simulink library "sf_aircraft_screen_library"  (Simulink 7.6)
settings: Solver=ode45  SolverMode=SingleTasking  StartTime=0.0  StopTime=10.0  RelTol=1e-3
settings Model: Creator=The MathWorks Inc.

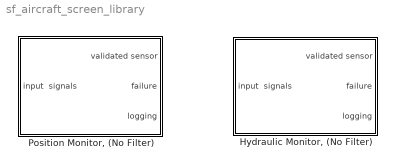
== system sf_aircraft_screen_library ==
  "Hydraulic Monitor, (No Filter)" : Subsystem  AncestorBlock=screen_library/Hydraulic Monitor
  "Position Monitor, (No Filter)" : Subsystem

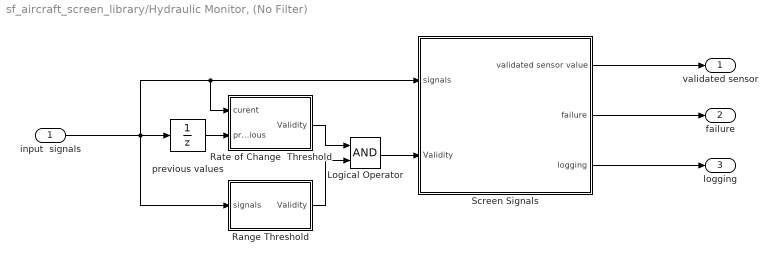
== system sf_aircraft_screen_library/Hydraulic Monitor, (No Filter) ==
  input  signals : Inport  PortDimensions=3  SampleTime=0.01
  Logical Operator : Logic  AllPortsSameDT=off
  Range Threshold : Subsystem
  Rate of Change  Threshold : Subsystem
  Screen Signals : Subsystem
  previous values : UnitDelay  SampleTime=-1
  validated sensor : Outport
  failure : Outport  Port=2
  logging : Outport  Port=3
  wires:
  Screen Signals/3(logging) -> logging/1
  Logical Operator/1 -> Screen Signals/2(Validity)
  Rate of Change  Threshold/1(Validity) -> Logical Operator/1
  Range Threshold/1(Validity) -> Logical Operator/2
  previous values/1 -> Rate of Change  Threshold/2(previous)
  Screen Signals/1(validated sensor value) -> validated sensor/1
  input  signals/1 -> Range Threshold/1(signals), Screen Signals/1(signals), Rate of Change  Threshold/1(curent), previous values/1
  Screen Signals/2(failure) -> failure/1

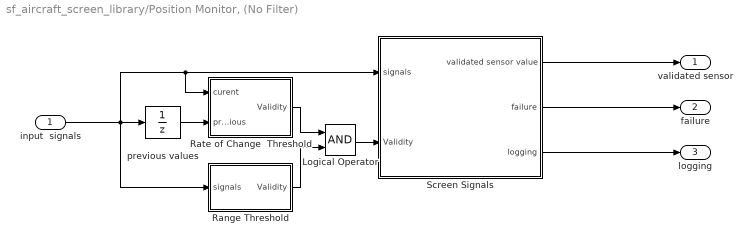
== system sf_aircraft_screen_library/Position Monitor, (No Filter) ==
  input  signals : Inport  PortDimensions=3  SampleTime=0.01
  Logical Operator : Logic  AllPortsSameDT=off
  Range Threshold : Subsystem  RequirementInfo={'other' 'Position Sensor Logic Requirements.doc' 'Out of Bound Readings' 'true' 'Out of Bound Readings' '' }
  Rate of Change  Threshold : Subsystem  RequirementInfo={'other' 'Position Sensor Logic Requirements.doc' 'Rate of Change of Readings' 'true' 'Rate of Change of Readings' '' }
  Screen Signals : Subsystem
  previous values : UnitDelay  SampleTime=-1
  validated sensor : Outport
  failure : Outport  Port=2
  logging : Outport  Port=3
  wires:
  Screen Signals/3(logging) -> logging/1
  Screen Signals/2(failure) -> failure/1
  input  signals/1 -> Range Threshold/1(signals), previous values/1, Screen Signals/1(signals), Rate of Change  Threshold/1(curent)
  Screen Signals/1(validated sensor value) -> validated sensor/1
  previous values/1 -> Rate of Change  Threshold/2(previous)
  Range Threshold/1(Validity) -> Logical Operator/2
  Rate of Change  Threshold/1(Validity) -> Logical Operator/1
  Logical Operator/1 -> Screen Signals/2(Validity)

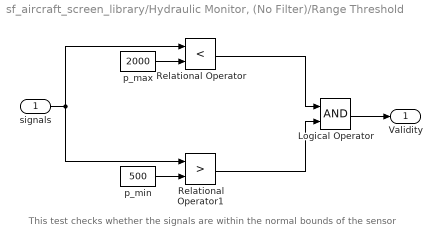
== system sf_aircraft_screen_library/Hydraulic Monitor, (No Filter)/Range Threshold ==
  note: This test checks whether the signals are within
      | the normal bounds of the sensor
  signals : Inport
  Logical Operator : Logic  AllPortsSameDT=off
  Relational Operator : RelationalOperator  Operator=<
  Relational Operator1 : RelationalOperator  Operator=>
  p_max : Constant  Value=2000
  p_min : Constant  Value=500
  Validity : Outport
  wires:
  Logical Operator/1 -> Validity/1
  p_min/1 -> Relational Operator1/2
  p_max/1 -> Relational Operator/2
  Relational Operator1/1 -> Logical Operator/2
  Relational Operator/1 -> Logical Operator/1
  signals/1 -> Relational Operator1/1, Relational Operator/1

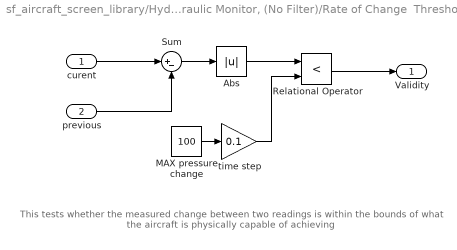
== system sf_aircraft_screen_library/Hydraulic Monitor, (No Filter)/Rate of Change  Threshold ==
  note: This tests whether the measured change between two readings
      | is within the bounds of what the aircraft is physically capable of achieving
  curent : Inport
  previous : Inport  Port=2
  Abs : Abs  SaturateOnIntegerOverflow=on
  MAX pressure change : Constant  Value=100
  Relational Operator : RelationalOperator  Operator=<  OutDataTypeStr=boolean
  Sum : Sum  Inputs=|+-  SaturateOnIntegerOverflow=on
  time step : Gain  Gain=0.1  SaturateOnIntegerOverflow=on  OutDataTypeStr=Inherit: Same as input  ParamDataTypeStr=Inherit: Same as input
  Validity : Outport
  wires:
  Sum/1 -> Abs/1
  time step/1 -> Relational Operator/2
  MAX pressure change/1 -> time step/1
  Relational Operator/1 -> Validity/1
  previous/1 -> Sum/2
  curent/1 -> Sum/1
  Abs/1 -> Relational Operator/1

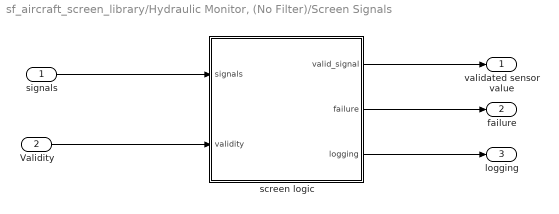
== system sf_aircraft_screen_library/Hydraulic Monitor, (No Filter)/Screen Signals ==
  signals : Inport
  Validity : Inport  Port=2
  screen logic : Stateflow chart  AncestorBlock=new_screening/Montior/Screen Signals/screen logic  TreatAsAtomicUnit=on
  validated sensor value : Outport
  failure : Outport  Port=2
  logging : Outport  Port=3
  wires:
  screen logic/3(logging) -> logging/1
  signals/1 -> screen logic/1(signals)
  Validity/1 -> screen logic/2(validity)
  screen logic/1(valid_signal) -> validated sensor value/1
  screen logic/2(failure) -> failure/1

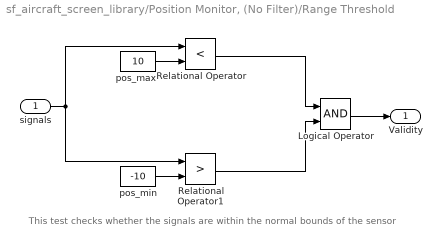
== system sf_aircraft_screen_library/Position Monitor, (No Filter)/Range Threshold ==
  note: This test checks whether the signals are within
      | the normal bounds of the sensor
  signals : Inport
  Logical Operator : Logic  AllPortsSameDT=off
  Relational Operator : RelationalOperator  Operator=<
  Relational Operator1 : RelationalOperator  Operator=>
  pos_max : Constant  Value=10
  pos_min : Constant  Value=-10
  Validity : Outport
  wires:
  Logical Operator/1 -> Validity/1
  pos_min/1 -> Relational Operator1/2
  pos_max/1 -> Relational Operator/2
  Relational Operator1/1 -> Logical Operator/2
  Relational Operator/1 -> Logical Operator/1
  signals/1 -> Relational Operator1/1, Relational Operator/1

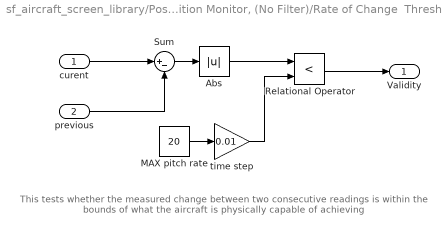
== system sf_aircraft_screen_library/Position Monitor, (No Filter)/Rate of Change  Threshold ==
  note: This tests whether the measured change between two consecutive readings
      | is within the bounds of what the aircraft is physically capable of achieving
  curent : Inport
  previous : Inport  Port=2
  Abs : Abs  SaturateOnIntegerOverflow=on
  MAX pitch rate : Constant  Value=20
  Relational Operator : RelationalOperator  Operator=<  OutDataTypeStr=boolean
  Sum : Sum  Inputs=|+-  SaturateOnIntegerOverflow=on
  time step : Gain  Gain=0.01  SaturateOnIntegerOverflow=on  OutDataTypeStr=Inherit: Same as input  ParamDataTypeStr=Inherit: Same as input
  Validity : Outport
  wires:
  curent/1 -> Sum/1
  previous/1 -> Sum/2
  Relational Operator/1 -> Validity/1
  MAX pitch rate/1 -> time step/1
  time step/1 -> Relational Operator/2
  Sum/1 -> Abs/1
  Abs/1 -> Relational Operator/1

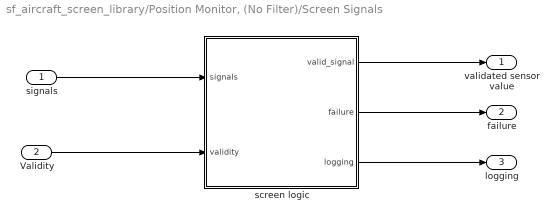
== system sf_aircraft_screen_library/Position Monitor, (No Filter)/Screen Signals ==
  signals : Inport
  Validity : Inport  Port=2
  screen logic : Stateflow chart  TreatAsAtomicUnit=on
  validated sensor value : Outport
  failure : Outport  Port=2
  logging : Outport  Port=3
  wires:
  screen logic/3(logging) -> logging/1
  screen logic/2(failure) -> failure/1
  screen logic/1(valid_signal) -> validated sensor value/1
  Validity/1 -> screen logic/2(validity)
  signals/1 -> screen logic/1(signals)

== stateflow chart Position Monitor, (No Filter)/Screen Signals/screen logic ==
  state num = valid_sensors() [function]
    (default) -> (junction 45)
    (junction 45) -> (junction 46) : { aVarTruthTableCondition_1 = (validity[1] == 1); }
    (junction 46) -> (junction 47) : { aVarTruthTableCondition_2 = (validity[2] == 1); }
    (junction 47) -> (junction 48) : { aVarTruthTableCondition_3 = (validity[3] == 1); }
    (junction 48) -> (junction 49) [order 1] : [aVarTruthTableCondition_1 && aVarTruthTableCondition_2 && aVarTruthTableCondition_3]
    (junction 49) -> (junction 50) : {
        | /* All 3 signals valid */
        | num = 3;
        | }
    (junction 48) -> (junction 51) [order 2]
    (junction 51) -> (junction 52) [order 1] : [aVarTruthTableCondition_1 && aVarTruthTableCondition_2 && !aVarTruthTableCondition_3]
    (junction 52) -> (junction 53) : {
        | /* Signals 1&2 valid */
        | num = 2;
        | select[1]=1;
        | select[2]=2;
        | }
    (junction 51) -> (junction 54) [order 2]
    (junction 54) -> (junction 55) [order 1] : [aVarTruthTableCondition_1 && !aVarTruthTableCondition_2 && aVarTruthTableCondition_3]
    (junction 55) -> (junction 56) : {
        | /* Signals 1&3 valid */
        | num = 2;
        | select[1]=1;
        | select[2]=3;
        | }
    (junction 54) -> (junction 57) [order 2]
    (junction 57) -> (junction 58) [order 1] : [aVarTruthTableCondition_1 && !aVarTruthTableCondition_2 && !aVarTruthTableCondition_3]
    (junction 58) -> (junction 59) : {
        | /* Signal 1 valid */
        | num = 1;
        | select[1]=1;
        | select[2]=0;
        | }
    (junction 57) -> (junction 60) [order 2]
    (junction 60) -> (junction 61) [order 1] : [!aVarTruthTableCondition_1 && aVarTruthTableCondition_2 && aVarTruthTableCondition_3]
    (junction 61) -> (junction 62) : {
        | /* Signals 2&3 valid */
        | num = 2;
        | select[1]=2;
        | select[2]=3;
        | }
    (junction 60) -> (junction 63) [order 2]
    (junction 63) -> (junction 64) [order 1] : [!aVarTruthTableCondition_1 && aVarTruthTableCondition_2 && !aVarTruthTableCondition_3]
    (junction 64) -> (junction 65) : {
        | /* Signal 2 valid */
        | num = 1;
        | select[1]=2;
        | select[2]=0;
        | }
    (junction 63) -> (junction 66) [order 2]
    (junction 66) -> (junction 67) [order 1] : [!aVarTruthTableCondition_1 && !aVarTruthTableCondition_2 && aVarTruthTableCondition_3]
    (junction 67) -> (junction 68) : {
        | /* Signal 3 valid */
        | num = 1;
        | select[1]=3;
        | select[2]=0;
        | }
    (junction 66) -> (junction 69) [order 2]
    (junction 69) -> (junction 70) [order 1] : [!aVarTruthTableCondition_1 && !aVarTruthTableCondition_2 && !aVarTruthTableCondition_3]
    (junction 70) -> (junction 71) : {
        | /* 'None':no signals valid */
        | num = 0;
        | }
    (junction 69) -> (junction 72) [order 2]
  state none() [function]
    (junction 22) -> (junction 21) [order 2] : {valid_signal=prev_signal;}
    (junction 21) -> (junction 27) : {failure=0;}
    (junction 20) -> (junction 36) : {failure=1;}
    (junction 23) -> (junction 20) : {valid_signal=0;}
    (junction 22) -> (junction 35) [order 1] : [count>3]
    (junction 24) -> (junction 22) : {count=count+1;}
    (default) -> (junction 24)
    (junction 27) -> (junction 36) : {send(log,failure_logging)}
    (junction 35) -> (junction 23) : {count=3;}
  state Screen [parallel]
    settings: executionOrder=1
    state zero
      (default) -> (junction 30) : {none();}
    state three
      (default) -> (junction 17) : {sum=signals[1]+signals[2]+signals[3];}
      (junction 34) -> (junction 16) [order 2] : {valid_signal=middle;}
      (junction 16) -> (junction 18) : {failure=0;}
      (junction 18) -> (junction 19) : {prev_signal=valid_signal;}
      (junction 34) -> (junction 40) [order 1] : [bad==1]
      (junction 19) -> (junction 39) : {count=0;}
      (junction 17) -> (junction 34) : {middle=sum-...
          | max(max(signals[1],signals[2]),signals[3])-...
          | min(min(signals[1],signals[2]),signals[3]);}
      (junction 40) -> (junction 31) : {none();}
    state two
      (junction 25) -> (junction 37) : {count=0;}
      (junction 28) -> (junction 26) : {failure=0;}
      (junction 29) -> (junction 28) : {valid_signal=mean;}
      (junction 26) -> (junction 25) : {prev_signal=valid_signal;}
      (junction 33) -> (junction 29) [order 2] : {mean=(signals[select[1]]+signals[select[2]])/2;}
      (junction 33) -> (junction 38) [order 1] : [diff>diff_max]
      (default) -> (junction 33) : {diff=abs(signals[select[1]]-signals[select[2]]);}
      (junction 38) -> (junction 32) : {none();}
    state one
      note: Only one valid sensor - just use the valid signal.
          | Failure is false
      (junction 42) -> (junction 43) : {failure=0;}
      (junction 43) -> (junction 44) : {prev_signal=valid_signal;}
      (junction 44) -> (junction 41) : {count=0;}
      (default) -> (junction 42) : {valid_signal=signals[select[1]];}
    note: no valid signals
    (default) -> (junction 15) : {n=valid_sensors();}
    zero -> Screen
    (junction 15) -> one [order 3] : [n==1]
    (junction 15) -> zero [order 4]
    (junction 15) -> three [order 1] : [n==3]
    (junction 15) -> two [order 2] : [n==2]
    two -> Screen
    three -> Screen
    one -> Screen
  state failure_logging [parallel]
    settings: executionOrder=2
    state off
    state logging
    (default) -> off
    logging -> off [order 1] : after(30,tick)[~failure]
    off -> logging : log
    logging -> logging [order 2] : log
  data: num function_output int8; aVarTruthTableCondition_1 temporary boolean =0; aVarTruthTableCondition_2 temporary boolean =0; aVarTruthTableCondition_3 temporary boolean =0; middle local double; sum local double; diff local double; mean local double; signals input double size=3; validity input boolean size=3; n local int8; valid_signal output double; failure output boolean; prev_signal local double; count local int8; diff_max constant double =3; bad local boolean; select local int8 size=2; logging output unknown
  events: log local EITHER_EDGE_EVENT

== stateflow chart Hydraulic Monitor, (No Filter)/Screen Signals/screen logic ==
  state num = valid_sensors() [function]
    (default) -> (junction 208)
    (junction 208) -> (junction 209) : { aVarTruthTableCondition_1 = (validity[1] == 1); }
    (junction 209) -> (junction 210) : { aVarTruthTableCondition_2 = (validity[2] == 1); }
    (junction 210) -> (junction 211) : { aVarTruthTableCondition_3 = (validity[3] == 1); }
    (junction 211) -> (junction 212) [order 1] : [aVarTruthTableCondition_1 && aVarTruthTableCondition_2 && aVarTruthTableCondition_3]
    (junction 212) -> (junction 213) : {
        | /* All 3 signals valid */
        | num = 3;
        | }
    (junction 211) -> (junction 214) [order 2]
    (junction 214) -> (junction 215) [order 1] : [aVarTruthTableCondition_1 && aVarTruthTableCondition_2 && !aVarTruthTableCondition_3]
    (junction 215) -> (junction 216) : {
        | /* Signals 1&2 valid */
        | num = 2;
        | select[1]=1;
        | select[2]=2;
        | }
    (junction 214) -> (junction 217) [order 2]
    (junction 217) -> (junction 218) [order 1] : [aVarTruthTableCondition_1 && !aVarTruthTableCondition_2 && aVarTruthTableCondition_3]
    (junction 218) -> (junction 219) : {
        | /* Signals 1&3 valid */
        | num = 2;
        | select[1]=1;
        | select[2]=3;
        | }
    (junction 217) -> (junction 220) [order 2]
    (junction 220) -> (junction 221) [order 1] : [aVarTruthTableCondition_1 && !aVarTruthTableCondition_2 && !aVarTruthTableCondition_3]
    (junction 221) -> (junction 222) : {
        | /* Signal 1 valid */
        | num = 1;
        | select[1]=1;
        | select[2]=0;
        | }
    (junction 220) -> (junction 223) [order 2]
    (junction 223) -> (junction 224) [order 1] : [!aVarTruthTableCondition_1 && aVarTruthTableCondition_2 && aVarTruthTableCondition_3]
    (junction 224) -> (junction 225) : {
        | /* Signals 2&3 valid */
        | num = 2;
        | select[1]=2;
        | select[2]=3;
        | }
    (junction 223) -> (junction 226) [order 2]
    (junction 226) -> (junction 227) [order 1] : [!aVarTruthTableCondition_1 && aVarTruthTableCondition_2 && !aVarTruthTableCondition_3]
    (junction 227) -> (junction 228) : {
        | /* Signal 2 valid */
        | num = 1;
        | select[1]=2;
        | select[2]=0;
        | }
    (junction 226) -> (junction 229) [order 2]
    (junction 229) -> (junction 230) [order 1] : [!aVarTruthTableCondition_1 && !aVarTruthTableCondition_2 && aVarTruthTableCondition_3]
    (junction 230) -> (junction 231) : {
        | /* Signal 3 valid */
        | num = 1;
        | select[1]=3;
        | select[2]=0;
        | }
    (junction 229) -> (junction 232) [order 2]
    (junction 232) -> (junction 233) [order 1] : [!aVarTruthTableCondition_1 && !aVarTruthTableCondition_2 && !aVarTruthTableCondition_3]
    (junction 233) -> (junction 234) : {
        | /* 'None':no signals valid */
        | num = 0;
        | }
    (junction 232) -> (junction 235) [order 2]
  state none() [function]
    (junction 184) -> (junction 183) : {count=3;}
    (junction 190) -> (junction 199) : {count=count+1;}
    (junction 199) -> (junction 184) [order 1] : [count>3]
    (junction 183) -> (junction 186) : {valid_signal=0;}
    (junction 199) -> (junction 185) [order 2] : {valid_signal=prev_signal;}
    (junction 185) -> (junction 198) : {failure=0;}
    (default) -> (junction 190)
    (junction 198) -> (junction 187) : {send(log,failure_logging)}
    (junction 186) -> (junction 187) : {failure=1;}
  state Screen [parallel]
    settings: executionOrder=1
    state one
      note: Only one valid sensor - just use the valid signal.
          | Failure is false
      (junction 205) -> (junction 193) : {prev_signal=valid_signal;}
      (default) -> (junction 206) : {valid_signal=signals[select[1]];}
      (junction 206) -> (junction 205) : {failure=0;}
      (junction 193) -> (junction 202) : {count=0;}
    state three
      (junction 201) -> (junction 204) : {count=0;}
      (junction 196) -> (junction 201) : {prev_signal=valid_signal;}
      (junction 195) -> (junction 196) : {failure=0;}
      (junction 191) -> (junction 195) [order 2] : {valid_signal=middle;}
      (junction 189) -> (junction 192) : {none();}
      (junction 188) -> (junction 191) : {middle=sum-...
          | max(max(signals[1],signals[2]),signals[3])-...
          | min(min(signals[1],signals[2]),signals[3]);}
      (default) -> (junction 188) : {sum=signals[1]+signals[2]+signals[3];}
      (junction 191) -> (junction 189) [order 1] : [bad==1]
    state two
      (junction 180) -> (junction 178) : {count=0;}
      (junction 182) -> (junction 179) : {none();}
      (junction 181) -> (junction 182) [order 1] : [diff>diff_max]
      (junction 197) -> (junction 203) : {failure=0;}
      (junction 194) -> (junction 197) : {valid_signal=mean;}
      (junction 181) -> (junction 194) [order 2] : {mean=(signals[select[1]]+signals[select[2]])/2;}
      (junction 203) -> (junction 180) : {prev_signal=valid_signal;}
      (default) -> (junction 181) : {diff=abs(signals[select[1]]-signals[select[2]]);}
    note: no valid signals
    state zero
      (default) -> (junction 207) : {none();}
    (default) -> (junction 200) : {n=valid_sensors();}
    (junction 200) -> zero [order 4]
    (junction 200) -> three [order 1] : [n==3]
    three -> Screen
    (junction 200) -> two [order 2] : [n==2]
    two -> Screen
    (junction 200) -> one [order 3] : [n==1]
    one -> Screen
    zero -> Screen
  state failure_logging [parallel]
    settings: executionOrder=2
    state logging
    state off
    logging -> off [order 1] : after(30,tick)[~failure]
    (default) -> off
    off -> logging : log
    logging -> logging [order 2] : log
  data: num function_output int8; aVarTruthTableCondition_1 temporary boolean =0; aVarTruthTableCondition_2 temporary boolean =0; aVarTruthTableCondition_3 temporary boolean =0; middle local double; sum local double; diff local double; mean local double; signals input double size=3; validity input boolean size=3; n local int8; valid_signal output double; failure output boolean; prev_signal local double; count local int8; diff_max constant double =10; bad local boolean; select local int8 size=2; logging output unknown
  events: log local EITHER_EDGE_EVENT
